simulink subsystem "PieroControlado1mz"  (R2023b)
settings: Solver=VariableStepAuto  StartTime=0.0  StopTime=10.0  RelTol=1e-3
undefined symbols (not defined in the file): DiscIntNeverNeededParam
settings Model: Creator=adria  LastModifiedBy=adria

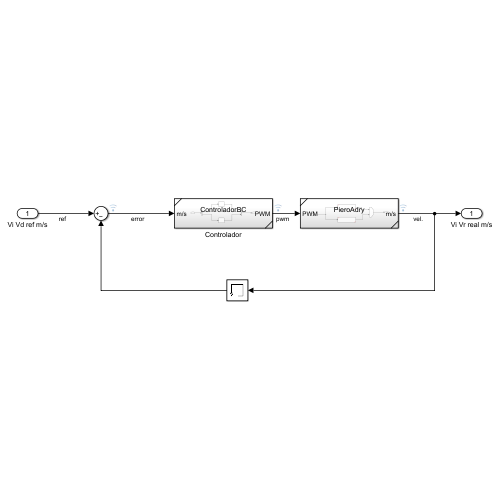
[thumbnail: Simulink's stored preview of the top-level diagram]
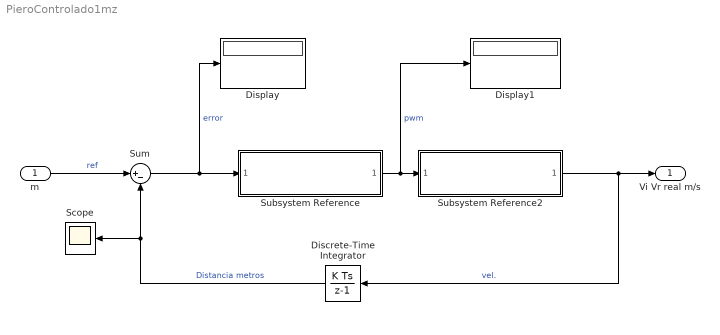
== system PieroControlado1mz ==
  m : Inport  OutDataTypeStr=double  PortDimensions=2
  Discrete-Time Integrator : DiscreteIntegrator  SampleTime=-1  ICPrevOutput=DiscIntNeverNeededParam  ICPrevScaledInput=DiscIntNeverNeededParam
  Display : Display
  Display1 : Display
  Scope : Scope
  Subsystem Reference : Subsystem  ReferencedSubsystem=ControladorPos1mz
  Subsystem Reference2 : Subsystem  ReferencedSubsystem=PieroAdryZ
  Sum : Sum  Inputs=|+-
  Vi Vr real m/s : Outport  OutDataTypeStr=double  PortDimensions=2
  wires:
  Subsystem Reference2/1 -> Vi Vr real m/s/1, Discrete-Time Integrator/1  "vel."
  Subsystem Reference/1 -> Subsystem Reference2/1, Display1/1  "pwm"
  m/1 -> Sum/1  "ref"
  Discrete-Time Integrator/1 -> Sum/2, Scope/1  "Distancia metros"
  Sum/1 -> Subsystem Reference/1, Display/1  "error"
